simulink model "P1_Ex5"  (R2018a)
settings: Solver=FixedStepAuto  StartTime=0.0  StopTime=20  RelTol=1e-3
PreLoadFcn:
  | % Sampling times
  | Tg=0.005;
  | Ts=0.01;
  | % Motor limits
  | Vmax=5;
  | Vmin=-5;
  | % Proportional controller's gain
  | Kp=1;
libraries: arduinolib x2, simulink x1
settings Model: SimulationMode=external  ExtModeTrigDuration=2  Creator=Eneko Lerma  LastModifiedBy=Eneko Lerma
settings OptimizationCC: EnhancedBackFolding=on  PassReuseOutputArgsAs=Individual arguments  MaxStackSize=64  OptimizeBlockOrder=speed  DifferentSizesBufferReuse=on  OptimizationCustomize=off
settings DebuggingCC: ParameterPrecisionLossMsg=none  ParameterTunabilityLossMsg=error
settings HardwareCC: ProdBitPerPointer=32  ProdBitPerSizeT=32  ProdBitPerPtrDiffT=32  ProdLargestAtomicInteger=Long  ProdLargestAtomicFloat=Double  ProdWordSize=32  ProdHWDeviceType=ARM Compatible->ARM Cortex
settings SFSimCC: MATLABDynamicMemAlloc=off
settings RTWCC: SystemTargetFile=ert.tlc  HardwareBoard=Arduino Due  TLCOptions=-aInlineSetEventsForThisBaseRateFcn=TLC_FALSE -aSuppressMultiTaskScheduler=TLC_FALSE -aRateBasedStepFcn=1  TemplateMakefile=ert_default_tmf  GenerateReport=on  Toolchain=Arduino ARM  BuildConfiguration=Faster Runs  IncludeHyperlinkInReport=on  LaunchReport=on  GenerateTraceInfo=on  GenerateTraceReport=on  GenerateTraceReportSl=on  GenerateTraceReportSf=on  GenerateTraceReportEml=on
settings CodeAppCC: ForceParamTrailComments=on  IgnoreCustomStorageClasses=off  OperatorAnnotations=on  SimulinkDataObjDesc=on  SFDataObjDesc=on  InsertBlockDesc=on
settings ERTTargetCC: SupportContinuousTime=on  SupportVariableSizeSignals=on

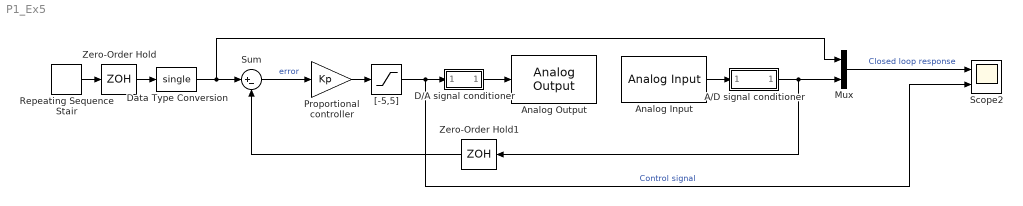
== system P1_Ex5 ==
  A/D signal conditioner : Subsystem
  Analog Input : arduinolib/Analog Input  pinNumber=2  ReadResultsOnly=off  ConversionTriggerSource=Software  ExternalTriggerType=uint32(0)  OutputDataType=uint16  EnableConversionCompleteNotify=off  EnableOuputStatus=off  SampleTime=Tg  blockPlatform=arduino
  Analog Output : arduinolib/Analog Output  DACpin=DAC1  blockPlatform=arduino
      settings: SourceProductName=Simulink Support Package for Arduino Hardware  SourceProductBaseCode=ARDUINO
  D/A signal conditioner : Subsystem
  Data Type Conversion : DataTypeConversion  OutDataTypeStr=single
  Mux : Mux  Inputs=2
  Proportional controller : Gain  Gain=Kp  OutDataTypeStr=single
  Repeating Sequence Stair : simulink/Sources/Repeating Sequence Stair  OutValues=[0 1 3 -1 2].'  tsamp=3  OutMin=[]  OutMax=[]  OutDataTypeStr=double  OutputDataTypeScalingMode=double  OutDataType=fixdt(0,8)  ConRadixGroup=Best Precision: Vector-wise  OutScaling=2^-12
  Scope2 : Scope  NumInputPorts=2
  Sum : Sum  Inputs=|+-
  Zero-Order Hold : ZeroOrderHold  SampleTime=Ts
  Zero-Order Hold1 : ZeroOrderHold  SampleTime=Ts
  "[-5,5]" : Saturate  UpperLimit=Vmax  LowerLimit=Vmin
  wires:
  Mux/1 -> Scope2/1  "Closed loop response"
  Repeating Sequence Stair/1 -> Zero-Order Hold/1
  A/D signal conditioner/1(" ") -> Zero-Order Hold1/1, Mux/2
  Analog Input/1 -> A/D signal conditioner/1("  ")
  D/A signal conditioner/1(" ") -> Analog Output/1
  Sum/1 -> Proportional controller/1  "error"
  Proportional controller/1 -> "[-5,5]"/1
  "[-5,5]"/1 -> Scope2/2, D/A signal conditioner/1("  ")  "Control signal"
  Data Type Conversion/1 -> Sum/1, Mux/1
  Zero-Order Hold/1 -> Data Type Conversion/1
  Zero-Order Hold1/1 -> Sum/2

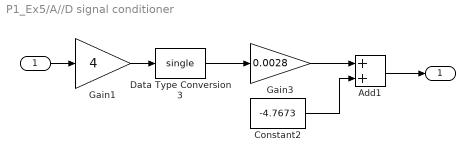
== system P1_Ex5/A//D signal conditioner ==
  "  " : Inport  OutDataTypeStr=uint16
  Add1 : Sum  AccumDataTypeStr=single
  Constant2 : Constant  Value=-4.7673  OutDataTypeStr=single
  Data Type Conversion3 : DataTypeConversion  OutDataTypeStr=single
  Gain1 : Gain  Gain=4  OutDataTypeStr=uint16
  Gain3 : Gain  Gain=0.0028  OutDataTypeStr=single
  " " : Outport  OutDataTypeStr=single
  wires:
  Gain1/1 -> Data Type Conversion3/1
  "  "/1 -> Gain1/1
  Data Type Conversion3/1 -> Gain3/1
  Gain3/1 -> Add1/1
  Constant2/1 -> Add1/2
  Add1/1 -> " "/1

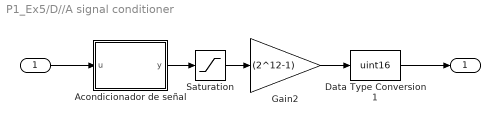
== system P1_Ex5/D//A signal conditioner ==
  "  " : Inport  OutDataTypeStr=single
  Acondicionador de señal : MATLAB Function  TreatAsAtomicUnit=on
  Data Type Conversion1 : DataTypeConversion  OutDataTypeStr=uint16
  Gain2 : Gain  Gain=(2^12-1)  OutDataTypeStr=single
  Saturation : Saturate  UpperLimit=1  LowerLimit=0  OutDataTypeStr=single
  " " : Outport  OutDataTypeStr=uint16
  wires:
  Gain2/1 -> Data Type Conversion1/1
  "  "/1 -> Acondicionador de señal/1(u)
  Acondicionador de señal/1(y) -> Saturation/1
  Data Type Conversion1/1 -> " "/1
  Saturation/1 -> Gain2/1

== matlab function P1_Ex5/D//A signal conditioner/Acondicionador de señal ==
  data: u input; y output
function y = fcn(u)
y =0.1342*u+0.3926;
